simulink model "function_call_test"  (Simulink 6.4)
settings: Solver=ode4  StartTime=0.0  StopTime=10  FixedStep=0.01  RelTol=1e-3
libraries: simulink x2, mpc_lib x1
settings Model: LastModifiedBy=Developer

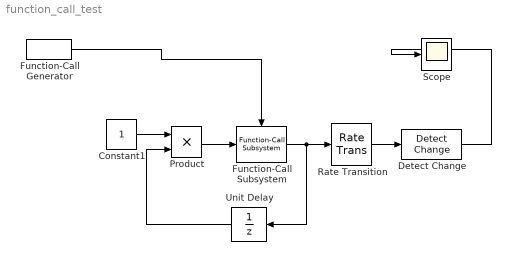
== system function_call_test ==
  Constant1 : Constant  Value=1  OutDataType=sfix(16)  ConRadixGroup=Use specified scaling  OutScaling=2^0  SampleTime=inf  FramePeriod=inf
  Detect Change : simulink/Logic and Bit Operations/Detect Change  SystemSampleTime=-1  vinit=1
  Function-Call Generator : simulink/Ports & Subsystems/Function-Call Generator  sample_time=1  numberOfIterations=100
  Function-Call Subsystem : mpc_lib/Subsystem/Function-Call Subsystem  SystemSampleTime=-1
  Product : Product  RndMeth=Zero
  Rate Transition : RateTransition  X0=1  OutPortSampleTime=0.02
  Scope : Scope
  Unit Delay : UnitDelay  Orientation=left  X0=1  SampleTime=-1
  wires:
  Function-Call Generator/1 -> Function-Call Subsystem/Trigger
  Function-Call Subsystem/1 -> Rate Transition/1, Unit Delay/1
  Constant1/1 -> Product/1
  Unit Delay/1 -> Product/2
  Product/1 -> Function-Call Subsystem/1
  Rate Transition/1 -> Detect Change/1
  Detect Change/1 -> Scope/1
